simulink model "Part4_Implementing_a_Simple_Vehicle_Lateral_Motion_1"  (R2021a)
settings: Solver=VariableStepAuto  StartTime=0.0  StopTime=100  RelTol=1e-3
libraries: vrlib x3, simulink x1, mpcadaslib x1
settings Model: Creator=QZHAN112  LastModifiedBy=QZHAN112

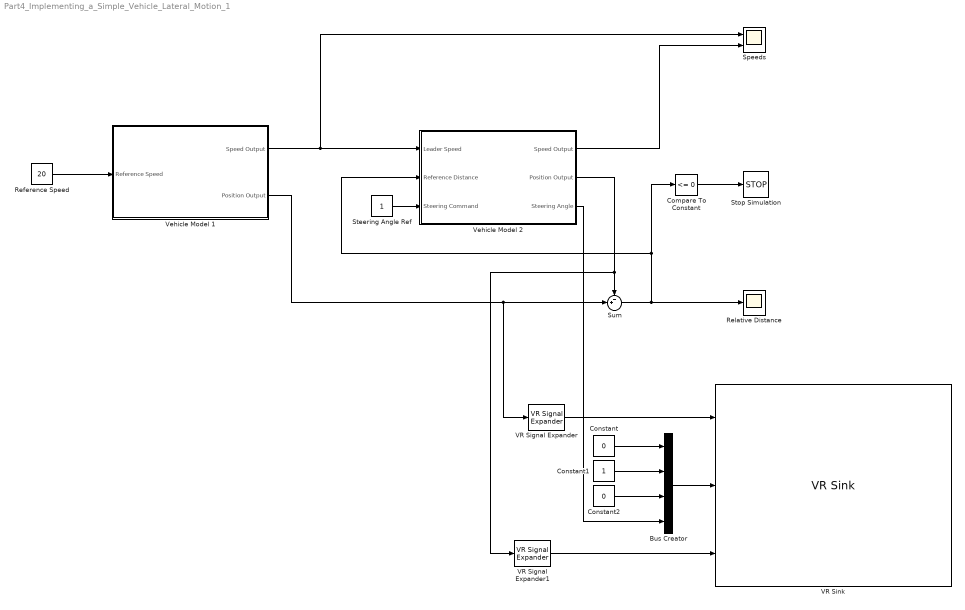
== system Part4_Implementing_a_Simple_Vehicle_Lateral_Motion_1 ==
  Bus Creator : BusCreator  Inputs=4
  Compare To Constant : simulink/Logic and Bit Operations/Compare To Constant  relop=<=  const=0  OutDataTypeStr=boolean
  Constant : Constant  Value=0
  Constant1 : Constant
  Constant2 : Constant  Value=0
  Reference Speed : Constant  Value=20
  Relative Distance : Scope
  Speeds : Scope  NumInputPorts=2
  Steering Angle Ref : Constant
  Stop Simulation : Stop
  Sum : Sum  Inputs=-+|
  VR Signal Expander : vrlib/VR Signal Expander  outwidth=3  outidx=[3]
  VR Signal Expander1 : vrlib/VR Signal Expander  outwidth=3  outidx=[3]
  VR Sink : vrlib/VR Sink  InstantiateOnLoad=on  SampleTime=0.05  ViewEnable=on  RemoteChange=off  RemoteView=off  FieldsWritten=Car_Red.translation.3.1.1.double#Car_Blue.rotation.4.1.1.double#Car_Blue.translation.3.1.1.double  WorldFileName=PlatoonWorld.WRL  AutoView=off  VideoDimensions=[]  AllowVariableSize=off  FigureProperties="{'Position', 'Name', 'Viewpoint', 'CameraBound', 'CameraDirection', 'CameraPosition', 'CameraUpVector', 'ZoomFactor', 'Antialiasing', 'Headlight', 'Lighting', 'NavPanel', 'Sound', 'StatusBar', 'Stereo3D', 'Stereo3DCameraOffset', 'Stereo3DHIT', 'ToolBar', 'Textures', 'Transparency', 'Triad', 'Wireframe', 'NavZones', 'NavMode', 'NavSpeed', 'CaptureFileFormat', 'CaptureFileName', 'Record2DCompressMethod', 'Record2DCompressQuality', 'Record2D', 'Record2DFileName', 'Record2DFPS'; [1.0000000000000000e+00   7.6000000000000000e+01   1.9200000000000000e+03   1.0330000000000000e+03], '', 'Cam_CarLotus', 'on', [0.0000000000000000e+00   0.0000000000000000e+00  -1.0000000000000000e+00], [0.0000000000000000e+00   0.0000000000000000e+00   0.0000000000000000e+00], [0.0000000000000000e+00   1.0000000000000000e+00   0.0000000000000000e+00], [1.0000000000000000e+00], 'on', 'on', 'on', 'halfbar', 'on', 'on', 'off', [1.0000000149011612e-01], [0.0000000000000000e+00], 'on', 'on', 'on', 'none', 'off', 'off', 'walk', 'normal', 'tif', '%f_anim_%n.tif', 'auto', [7.5000000000000000e+01], 'off', '%f_anim_%n.avi', 'auto'}"
  Vehicle Model 1 : Subsystem  mask{Pos=30, Speed=15}
      mask prompts: Pos "Initial Position"; Speed "Initial Speed"
      mask TypeOptions Pos: Initial Position/Value
      mask TypeOptions Speed: Initial Speed/Value
      mask Display: image('model-based autonomous traffic simulation framework\Scratch.jpg');
  Vehicle Model 2 : Subsystem  mask{Pos=0, Speed=30}
      mask prompts: Pos "Initial Position"; Speed "Initial Speed"
      mask TypeOptions Pos: Initial Position/Value
      mask TypeOptions Speed: Initial Speed/Value
      mask Display: image('model-based autonomous traffic simulation framework\Car-Design-Drawing-From-Shoulder.jpg');
  wires:
  Vehicle Model 1/2(Position Output) -> Sum/2, VR Signal Expander/1
  Reference Speed/1 -> Vehicle Model 1/1(Reference Speed)
  Vehicle Model 2/1(Speed Output) -> Speeds/2
  Vehicle Model 1/1(Speed Output) -> Speeds/1, Vehicle Model 2/1(Leader Speed)
  Sum/1 -> Compare To Constant/1, Vehicle Model 2/2(Reference Distance), Relative Distance/1
  Vehicle Model 2/2(Position Output) -> Sum/1, VR Signal Expander1/1
  Compare To Constant/1 -> Stop Simulation/1
  Steering Angle Ref/1 -> Vehicle Model 2/3(Steering Command)
  VR Signal Expander/1 -> VR Sink/1
  VR Signal Expander1/1 -> VR Sink/3
  Vehicle Model 2/3(Steering Angle) -> Bus Creator/4
  Bus Creator/1 -> VR Sink/2
  Constant/1 -> Bus Creator/1
  Constant1/1 -> Bus Creator/2
  Constant2/1 -> Bus Creator/3

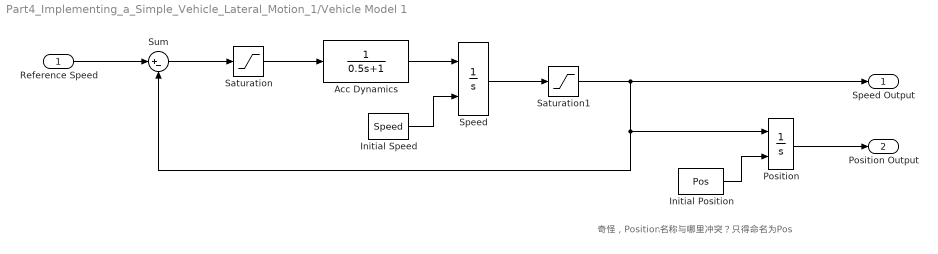
== system Part4_Implementing_a_Simple_Vehicle_Lateral_Motion_1/Vehicle Model 1 ==
  note: 奇怪，Position名称与哪里冲突？只得命名为Pos
  Reference Speed : Inport
  Acc Dynamics : TransferFcn  Denominator=[0.5 1]
  Initial Position : Constant  Value=Pos
  Initial Speed : Constant  Value=Speed
  Position : Integrator  InitialConditionSource=external
  Saturation : Saturate  UpperLimit=2  LowerLimit=-3
  Saturation1 : Saturate  UpperLimit=inf  LowerLimit=0
  Speed : Integrator  InitialConditionSource=external
  Sum : Sum  Inputs=|+-
  Speed Output : Outport
  Position Output : Outport  Port=2
  wires:
  Saturation/1 -> Acc Dynamics/1
  Acc Dynamics/1 -> Speed/1
  Speed/1 -> Saturation1/1
  Position/1 -> Position Output/1
  Saturation1/1 -> Speed Output/1, Sum/2, Position/1
  Reference Speed/1 -> Sum/1
  Initial Speed/1 -> Speed/2
  Sum/1 -> Saturation/1
  Initial Position/1 -> Position/2

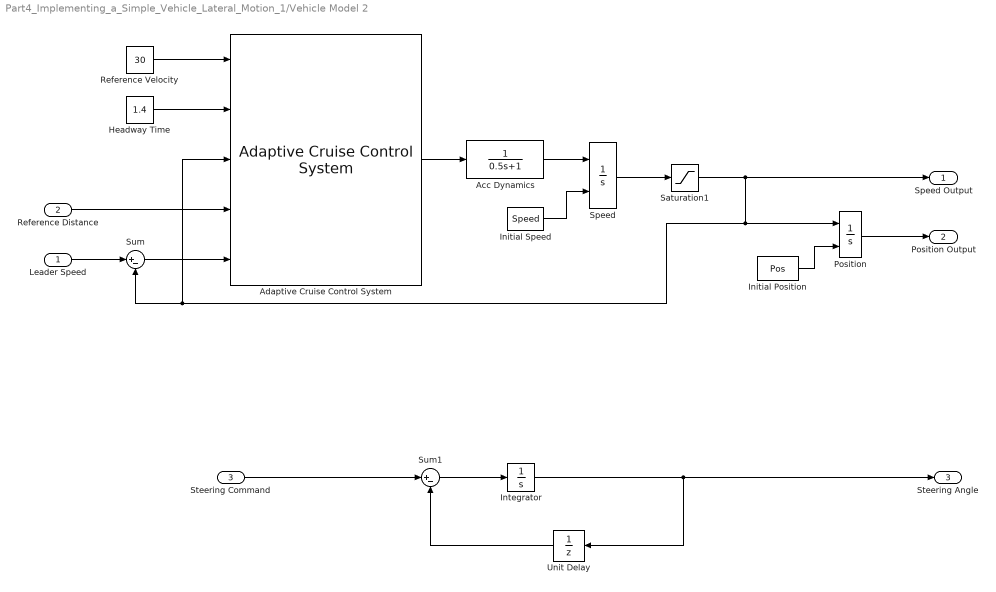
== system Part4_Implementing_a_Simple_Vehicle_Lateral_Motion_1/Vehicle Model 2 ==
  Leader Speed : Inport
  Reference Distance : Inport  Port=2
  Steering Command : Inport  Port=3
  Acc Dynamics : TransferFcn  Denominator=[0.5 1]
  Adaptive Cruise Control System : mpcadaslib/Adaptive Cruise Control System  EgoModel=tf(1,[0.5,1,0])  InitialEgoVelocity=30  DefaultSpacing=10  MaxVelocity=50  MinAcceleration=-3  amin_ext=off  MaxAcceleration=2  amax_ext=off  Ts=0.1  PredictionHorizon=300  ControllerBehavior=0.800  suboptimal=off  maxiter=10  datatypeopt=double  optmode=off  trackmode=off
  Headway Time : Constant  Value=1.4
  Initial Position : Constant  Value=Pos
  Initial Speed : Constant  Value=Speed
  Integrator : Integrator
  Position : Integrator  InitialConditionSource=external
  Reference Velocity : Constant  Value=30
  Saturation1 : Saturate  UpperLimit=inf  LowerLimit=0
  Speed : Integrator  InitialConditionSource=external
  Sum : Sum  Inputs=|+-
  Sum1 : Sum  Inputs=|+-
  Unit Delay : UnitDelay  SampleTime=-1  HasFrameUpgradeWarning=on
  Speed Output : Outport
  Position Output : Outport  Port=2
  Steering Angle : Outport  Port=3
  wires:
  Acc Dynamics/1 -> Speed/1
  Speed/1 -> Saturation1/1
  Position/1 -> Position Output/1
  Leader Speed/1 -> Sum/1
  Initial Speed/1 -> Speed/2
  Initial Position/1 -> Position/2
  Reference Distance/1 -> Adaptive Cruise Control System/4
  Headway Time/1 -> Adaptive Cruise Control System/2
  Reference Velocity/1 -> Adaptive Cruise Control System/1
  Sum/1 -> Adaptive Cruise Control System/5
  Adaptive Cruise Control System/1 -> Acc Dynamics/1
  Saturation1/1 -> Speed Output/1, Adaptive Cruise Control System/3, Sum/2, Position/1
  Sum1/1 -> Integrator/1
  Steering Command/1 -> Sum1/1
  Integrator/1 -> Unit Delay/1, Steering Angle/1
  Unit Delay/1 -> Sum1/2
